simulink model "case2_DCMG_attack_network_detailed_model_R2016"  (R2016a)
settings: Solver=FixedStepDiscrete  SolverMode=SingleTasking  StartTime=0.0  StopTime=3.5  FixedStep=Ts  RelTol=1e-3
InitFcn:
  | Ts=10e-6;
  | R1=0.5;
  | R2=0.6;
  | RD1=4;
  | RD2=4;
  | Vdc1=350;
  | Vdc2=350;
  | Vdcmg_ref=125;
  | Vc1_ref=125;
  | Vc2_ref=125;
model workspace (MAT data in the model file):
  Hamed_Najafi = 1
undefined symbols (not defined in the file): powergui, spspowerguiLib
libraries: powerlib x37, neural x15, simulink x6, powerlib_meascontrol x1
(part 1 of 2)
settings Model: Creator=Aminsystem  LastModifiedBy=Aminsystem
settings DataIOCC: SaveOutput=off  SignalLogging=off  DSMLogging=off  SaveTime=off
settings DebuggingCC: UnconnectedInputMsg=none  UnconnectedOutputMsg=none  UnconnectedLineMsg=none  SFUnexpectedBacktrackingDiag=error  SFNoUnconditionalDefaultTransitionDiag=error
settings ModelReferenceCC: EnableRefExpFcnMdlSchedulingChecks=off
settings SFSimCC: SimUseLocalCustomCode=on
settings RTWCC: Description=Generic Real-Time Target  RTWUseLocalCustomCode=on
settings GRTTargetCC: TargetLangStandard=C99 (ISO)
settings ConfigComp: CovMetricSettings=dwe  CovSaveCumulativeToWorkspaceVar=off  CovSaveSingleToWorkspaceVar=off  CovExternalEMLEnable=on

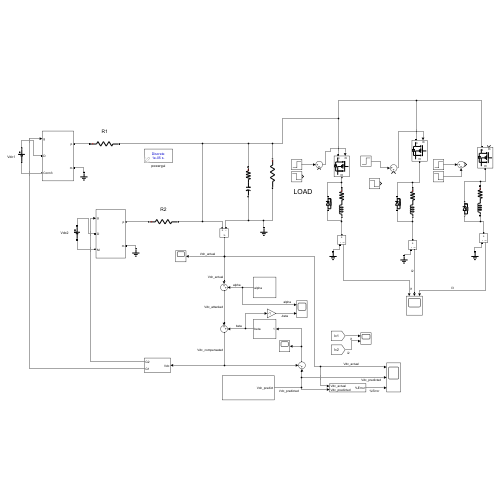
[thumbnail: Simulink's stored preview of the top-level diagram]
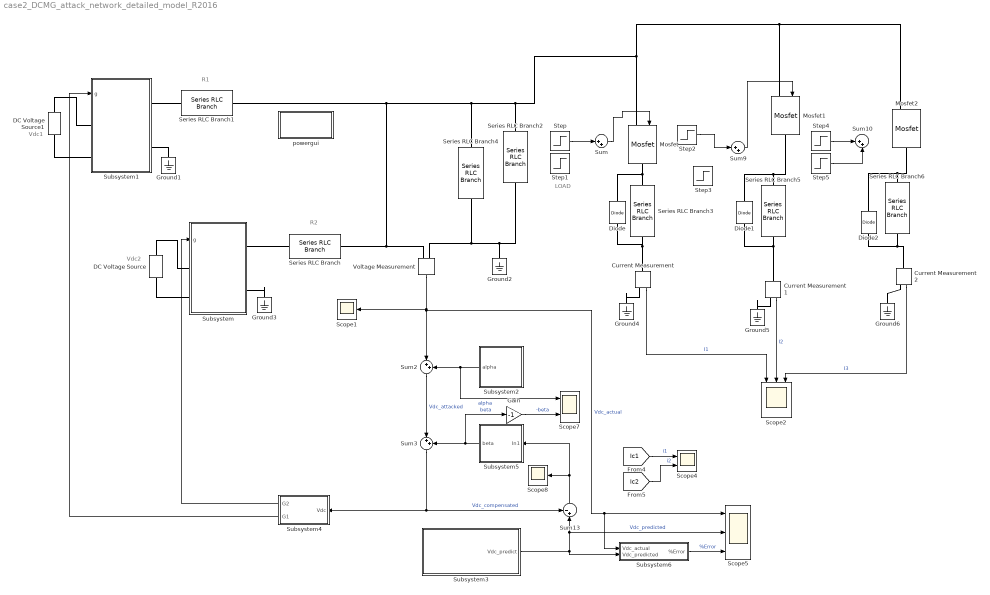
== system case2_DCMG_attack_network_detailed_model_R2016 ==
  note: Vdc2
  note: R2
  note: LOAD
  note: R1
  note: Vdc1
  Current Measurement : powerlib/Measurements/Current Measurement  PhasorSimulation=off  OutputType=Complex  PSBequivalent=0
  Current Measurement1 : powerlib/Measurements/Current Measurement  PhasorSimulation=off  OutputType=Complex  PSBequivalent=0
  Current Measurement2 : powerlib/Measurements/Current Measurement  PhasorSimulation=off  OutputType=Complex  PSBequivalent=0
  DC Voltage Source : powerlib/Electrical Sources/DC Voltage Source  Amplitude=Vdc2  Measurements=None
  DC Voltage Source1 : powerlib/Electrical Sources/DC Voltage Source  Amplitude=Vdc1  Measurements=None
  Diode : powerlib/Power Electronics/Diode  Ron=0.001  Lon=0  Vf=0.8  IC=0  UseSnubber=0  Rs=500  Cs=250e-9  Measurements=off
  Diode1 : powerlib/Power Electronics/Diode  Ron=0.001  Lon=0  Vf=0.8  IC=0  UseSnubber=0  Rs=500  Cs=250e-9  Measurements=off
  Diode2 : powerlib/Power Electronics/Diode  Ron=0.001  Lon=0  Vf=0.8  IC=0  UseSnubber=0  Rs=500  Cs=250e-9  Measurements=off
  Gain : Gain  Gain=-1
  Ground{1..6} (6 alike) : powerlib/Elements/Ground  LConnTagsString=a
  Mosfet : powerlib/Power Electronics/Mosfet  Ron=0.1  Lon=0  Rd=0.01  Vfd=0  IC=0  Rs=1e5  Cs=inf  Measurements=off
  Mosfet1 : powerlib/Power Electronics/Mosfet  Ron=0.1  Lon=0  Rd=0.01  Vfd=0  IC=0  Rs=1e5  Cs=inf  Measurements=off
  Mosfet2 : powerlib/Power Electronics/Mosfet  Ron=0.1  Lon=0  Rd=0.01  Vfd=0  IC=0  Rs=1e5  Cs=inf  Measurements=off
  Scope1 : Scope
  Scope2 : Scope  NumInputPorts=3
  Scope4 : Scope  NumInputPorts=2
  Scope5 : Scope  NumInputPorts=3
  Scope7 : Scope  NumInputPorts=2
  Scope8 : Scope
  Series RLC Branch : powerlib/Elements/Series RLC Branch  LConnTagsString=__new0  RConnTagsString=__new0  BranchType=R  Resistance=R2  Inductance=1e-3  SetiL0=off  InitialCurrent=0  Capacitance=1e-6  Setx0=off  InitialVoltage=0  Measurements=None
  Series RLC Branch1 : powerlib/Elements/Series RLC Branch  LConnTagsString=__new0  RConnTagsString=__new0  BranchType=R  Resistance=R1  Inductance=1e-3  SetiL0=off  InitialCurrent=0  Capacitance=1e-6  Setx0=off  InitialVoltage=0  Measurements=None
  Series RLC Branch2 : powerlib/Elements/Series RLC Branch  LConnTagsString=__new0  RConnTagsString=__new0  BranchType=R  Resistance=60  Inductance=1e-3  SetiL0=off  InitialCurrent=0  Capacitance=1e-6  Setx0=off  InitialVoltage=0  Measurements=None
  Series RLC Branch3 : powerlib/Elements/Series RLC Branch  LConnTagsString=__new0  RConnTagsString=__new0  BranchType=RL  Resistance=60  Inductance=2e-3  SetiL0=off  InitialCurrent=0  Capacitance=1e-6  Setx0=off  InitialVoltage=0  Measurements=None
  Series RLC Branch4 : powerlib/Elements/Series RLC Branch  LConnTagsString=__new0  RConnTagsString=__new0  BranchType=RC  Resistance=0.01  Inductance=1e-3  SetiL0=off  InitialCurrent=0  Capacitance=100e-6  Setx0=on  InitialVoltage=125  Measurements=None
  Series RLC Branch5 : powerlib/Elements/Series RLC Branch  LConnTagsString=__new0  RConnTagsString=__new0  BranchType=RL  Resistance=120  Inductance=5e-3  SetiL0=off  InitialCurrent=0  Capacitance=1e-6  Setx0=off  InitialVoltage=0  Measurements=None
  Series RLC Branch6 : powerlib/Elements/Series RLC Branch  LConnTagsString=__new0  RConnTagsString=__new0  BranchType=RL  Resistance=1.5  Inductance=10e-3  SetiL0=off  InitialCurrent=0  Capacitance=1e-6  Setx0=off  InitialVoltage=0  Measurements=None
  Step : Step  Time=0.5  SampleTime=Ts
  Step1 : Step  Time=2.3  After=-1  SampleTime=Ts
  Step2 : Step  Time=2.5  SampleTime=Ts
  Step3 : Step  Time=3.5  After=-1  SampleTime=Ts
  Step4 : Step  Time=4  SampleTime=Ts
  Step5 : Step  Time=4.2  After=-1  SampleTime=Ts
  Subsystem : Subsystem
  Subsystem1 : Subsystem
  Subsystem2 : Subsystem
  Subsystem3 : Subsystem
  Subsystem4 : Subsystem
  Subsystem5 : Subsystem
  Subsystem6 : Subsystem
  Sum{,2..3,9..10} (5 alike) : Sum  Inputs=|++
  Sum13 : Sum  Inputs=-+|
  Voltage Measurement : powerlib/Measurements/Voltage Measurement  PhasorSimulation=off  OutputType=Complex  PSBequivalent=0
  powergui : Subsystem  Priority=1  AncestorBlock=spspowerguiLib/powergui  DialogController=POWERSYS.PowerSysDialog  InitFcn=powergui( 'InitFcn_Callback' , gcb , 0 , [ ] );  mask(PSB option menu block){SimulationMode=Discrete, SampleTime=Ts, frequency=60, Iterations=50, frequencyindice=0, Pbase=100e6, ErrMax=1e-4, UnitsV=kV, UnitsW=MW, buscounter=0, FunctionMessages=off, echomessages=off, EnableUseOfTLC=off, CurrentSourceSwitches=off, DisableSnubberDevices=off, DisableRonSwitches=off, DisableVfSwitches=off, DisplayEquations=off, AutomaticDiscreteSolvers=off, SolverType=Tustin/Backward Euler (TBE), Interpol=off, ExternalGateDelay=off, methode=off, Ts=100, x0status=blocks, SPID=on, SwTol=0, HookPort=off, NonlinearTolerance=1e-4, nMaxIteration=100, ContinueOnMaxIteration=off, RestoreLinks=warning, ResistiveCurrentMeasurement=off, Frange=[0:2:500], Ylog=off, Xlog=on, ShowGrid=off, save=off, variable=ZData, structure=0, ZoomFFT=off, StartTime=0.0, cycles=1, DisplayStyle=1, fundamental=60, FreqAxis=off, MaxFrequency=1000, frequencyindicesteady=1, RmsSteady=1, display=off}
      mask prompts: SimulationMode "Simulation type:"; SampleTime "Sample time (s):"; frequency "Frequency (Hz):"; Iterations "Max iterations"; frequencyindice "Frequency (Hz)"; Pbase "Base power (VA)"; ErrMax "PQ tolerance (pu)"; UnitsV "Voltage units"; UnitsW "Power units"; buscounter "Load flow bus counter"; FunctionMessages "Disable Specialized Power Systems warnings"; echomessages "Display Specialized Power Systems compilation messages"; EnableUseOfTLC "Use TLC file when in Accelerator Simulation Mode and for code generation"; CurrentSourceSwitches "Disable ideal switching"; DisableSnubberDevices "Disable snubbers in switching devices"; DisableRonSwitches "Disable Ron resistances in switching devices"; DisableVfSwitches "Disable forward voltages in switching devices"; DisplayEquations "Display circuit differential equations"; AutomaticDiscreteSolvers "Automatically handle Discrete solver and Advanced tab solver settings of blocks"; SolverType "Discrete solver"; Interpol "Interpolate switching events"; ExternalGateDelay "Use time-stamped gate signals"; methode "Store switching topologies"; Ts "Buffer size (MBytes):"; x0status "Start simulation with initial electrical states from:"; SPID "Use ideal switching devices"; SwTol "Switch tolerance"; HookPort "Allow multiple powergui blocks"; NonlinearTolerance "Solver tolerance"; nMaxIteration "Maximum number of iterations"; ContinueOnMaxIteration "Continue Simulation if maximum number of iterations is reached"; RestoreLinks "Restore disabled links of Simscape Power Systems ST blocks:"; ResistiveCurrentMeasurement "Use non ideal current measurement blocks (1e-4Ohm internal resistance)"; Frange "Frequency Range"; Ylog "Log impedance"; Xlog "log Frequency"; ShowGrid "grid"; save "Save Data To Workspace"; variable "Variable Name"; structure "Structure Name (PSBFFTSCOPE)"; ZoomFFT "ZoomFFT (PSBFFTSCOPE)"; StartTime "Start Time (PSBFFTSCOPE)"; cycles "Cycles (PSBFFTSCOPE)"; DisplayStyle "Display style (PSBFFTSCOPE)"; fundamental "Fundamental (PSBFFTSCOPE)"; FreqAxis "Frequency Axis (PSBFFTSCOPE)"; MaxFrequency "Max Frequency (PSBFFTSCOPE)"; frequencyindicesteady "Frequency indice (STEADYSTATE)"; RmsSteady "RMS display (STEADYSTATE)"; display "Display Results"
      mask help: Set simulation type, simulation parameters, and preferences.
      mask init:
      | dispMessage = '';
      | dispMessage = powergui('MaskInitialization',gcb,SimulationMode,SampleTime);
      settings: PreSaveFcn=powergui( 'PreSaveFcn_Callback' , gcb , [ ] , [ ] );  OpenFcn=sps_rtmsupport('OpenFcn',gcbh)
      mask Help: helpview(psbhelp)
      mask TypeOptions SimulationMode: Continuous | Discrete | Phasor | Discrete phasor
      mask Callback SimulationMode: powergui('SimulationType',[],[],gcb);
      mask TypeOptions UnitsV: V | kV
      mask TypeOptions UnitsW: W | kW | MW
      mask Callback CurrentSourceSwitches: powergui('SimulationType',[],[],gcb);
      mask Callback AutomaticDiscreteSolvers: powergui('SimulationType',[],[],gcb);
      mask TypeOptions SolverType: Tustin/Backward Euler (TBE) | Tustin | Backward Euler
      mask Callback SolverType: powergui('SimulationType',[],[],gcb);
      mask Callback Interpol: powergui('SimulationType',[],[],gcb);
      mask Callback ExternalGateDelay: powergui('SimulationType',[],[],gcb);
      mask Callback methode: powergui('SimulationType',[],[],gcb);
      mask TypeOptions x0status: blocks | steady | zero
      mask TypeOptions RestoreLinks: yes | warning | no
      mask Callback display: sps_rtmsupport('parametereditingmodes',gcbh) % Will be executed last in parameter callbacks to ensure mask enable consistency
      mask DialogControl AutoSolverNote Prompt: The Simulation type parameter is governed by Simulink. To access the Powergui solver settings, unselect auto (Automatic solver selection) solver in the Simulink solver options.
      mask DialogControl StateAnalyzer Prompt: Measurements and States Analyzer
      mask DialogControl StateAnalyzer Callback: powerStates(bdroot(gcb))
      mask DialogControl LineParameterCalculator Prompt: Line Parameter Calculator
      mask DialogControl LineParameterCalculator Callback:
      | close_system(gcb)
      | powerLineParameters
      mask DialogControl CableParameterCalculator Prompt: Cable Parameter Calculator
      mask DialogControl CableParameterCalculator Callback:
      | close_system(gcb)
      | powerCableParameters
      mask DialogControl LineDecoupler Prompt: Line Decoupler
      mask DialogControl LineDecoupler Tooltip: Click to replace selected Distributed Parameters Line blocks with Decoupling Line blocks
      mask DialogControl LineDecoupler Callback:
      | close_system(gcb);
      | DecouplingLineReplace(gcs)
      mask DialogControl LoadFlowAnalyzer Prompt: Load Flow Analyzer
      mask DialogControl LoadFlowAnalyzer Callback:
      | close_system(gcb)
      | powerLoadFlow
      mask DialogControl LoadFlowParameters Prompt: Load Flow Parameters
      mask DialogControl ImpedanceCalculator Prompt: Impedance Calculator
      mask DialogControl ImpedanceCalculator Callback:
      | close_system(gcb);
      | powerImpedance(bdroot(gcs));
      mask DialogControl FFTAnalyzer Prompt: FFT Analyzer
      mask DialogControl FFTAnalyzer Callback:
      | close_system(gcb)
      | power_fftscope(bdroot(gcb),gcb)
      mask DialogControl LinearSystemAnalyzer Prompt: Linear System Analyzer
      mask DialogControl LinearSystemAnalyzer Callback:
      | close_system(gcb)
      | power_ltiview(bdroot(gcb))
      mask DialogControl HysteresisDesigner Prompt: Hysteresis Designer
      mask DialogControl HysteresisDesigner Callback:
      | close_system(gcb)
      | powerHysteresis('hysteresis.mat')
      mask DialogControl BlockCustomizer Prompt: Block Customizer
      mask DialogControl BlockCustomizer Callback:
      | close_system(gcb);
      | power_customize;
      mask DialogControl ReportGenerator Prompt: Report Generator
      mask DialogControl ReportGenerator Callback:
      | close_system(gcb)
      | power_report(bdroot(gcb))
      mask DialogControl obsolete Prompt: ...
      mask DialogControl MachineInitialization Prompt: Machine Initialization
      mask DialogControl MachineInitialization Callback:
      | close_system(gcb)
      | powericon('machineInitTool',bdroot(gcb),gcb)
      mask DialogControl Solver Prompt: Solver
      mask DialogControl SolverDetails Prompt: Solver details for nonlinear elements
      mask Display: color('blue'),disp(dispMessage)
  wires:
  Sum3/1 -> Sum13/1, Subsystem4/1(Vdc)  "Vdc_compensated"
  Step/1 -> Sum/1
  Sum/1 -> Mosfet/1
  Step2/1 -> Sum9/1
  Step4/1 -> Sum10/1
  Step5/1 -> Sum10/2
  Current Measurement/1 -> Scope2/1  "I1"
  Current Measurement1/1 -> Scope2/2  "I2"
  Current Measurement2/1 -> Scope2/3  "I3"
  Sum9/1 -> Mosfet1/1
  Voltage Measurement/1 -> Sum2/1, Scope5/1, Subsystem6/1(Vdc_actual), Scope1/1  "Vdc_actual"
  Sum13/1 -> Subsystem5/1(In1), Scope8/1
  [Ic1] -> Scope4/1  "i1"
  [Ic2] -> Scope4/2  "i2"
  Subsystem3/1(Vdc_predict) -> Scope5/2, Sum13/2, Subsystem6/2(Vdc_predicted)  "Vdc_predicted"
  Sum2/1 -> Sum3/1  "Vdc_attacked"
  Subsystem4/2(G1) -> Subsystem1/1(g)
  Subsystem4/1(G2) -> Subsystem/1(g)
  Subsystem2/1(alpha) -> Sum2/2, Scope7/1  "alpha"
  Subsystem5/1(beta) -> Gain/1, Sum3/2  "beta"
  Subsystem6/1(%Error) -> Scope5/3  "%Error"
  Gain/1 -> Scope7/2  "-beta"
  connections:
  Series RLC Branch5/RConn1 -- Diode1/LConn1 -- Current Measurement1/LConn1
  Series RLC Branch2/LConn1 -- Mosfet/LConn1 -- Mosfet2/LConn1 -- Mosfet1/LConn1 -- Series RLC Branch4/LConn1 -- Series RLC Branch1/RConn1 -- Series RLC Branch/RConn1 -- Voltage Measurement/LConn1
  Mosfet/RConn1 -- Diode/RConn1 -- Series RLC Branch3/LConn1
  Series RLC Branch3/RConn1 -- Diode/LConn1 -- Current Measurement/LConn1
  Voltage Measurement/LConn2 -- Ground2/LConn1 -- Series RLC Branch2/RConn1 -- Series RLC Branch4/RConn1
  Current Measurement2/LConn1 -- Diode2/LConn1 -- Series RLC Branch6/RConn1
  Series RLC Branch5/LConn1 -- Mosfet1/RConn1 -- Diode1/RConn1
  Diode2/RConn1 -- Mosfet2/RConn1 -- Series RLC Branch6/LConn1
  Series RLC Branch/LConn1 -- Subsystem/RConn1
  Subsystem/LConn1 -- DC Voltage Source/RConn1
  DC Voltage Source/LConn1 -- Subsystem/LConn2
  Series RLC Branch1/LConn1 -- Subsystem1/RConn1
  Subsystem1/LConn1 -- DC Voltage Source1/RConn1
  Subsystem1/LConn2 -- DC Voltage Source1/LConn1
  Ground1/LConn1 -- Subsystem1/RConn2
  Ground3/LConn1 -- Subsystem/RConn2
  Ground4/LConn1 -- Current Measurement/RConn1
  Ground5/LConn1 -- Current Measurement1/RConn1
  Ground6/LConn1 -- Current Measurement2/RConn1

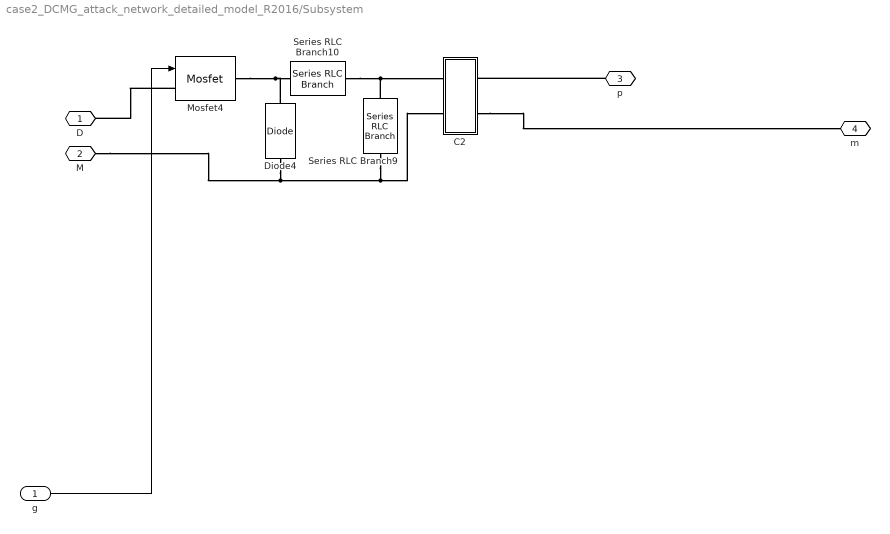
== system case2_DCMG_attack_network_detailed_model_R2016/Subsystem ==
  g : Inport
  C2 : Subsystem
  Diode4 : powerlib/Power Electronics/Diode  Ron=0.001  Lon=0  Vf=0.8  IC=0  UseSnubber=0  Rs=500  Cs=250e-9  Measurements=off
  Mosfet4 : powerlib/Power Electronics/Mosfet  Ron=0.1  Lon=0  Rd=0.01  Vfd=0  IC=0  Rs=1e5  Cs=inf  Measurements=off
  Series RLC Branch10 : powerlib/Elements/Series RLC Branch  LConnTagsString=__new0  RConnTagsString=__new0  BranchType=L  Resistance=0.01  Inductance=50e-3  SetiL0=off  InitialCurrent=0  Capacitance=57e-6  Setx0=off  InitialVoltage=120  Measurements=None
  Series RLC Branch9 : powerlib/Elements/Series RLC Branch  LConnTagsString=__new0  RConnTagsString=__new0  BranchType=C  Resistance=0.01  Inductance=1e-3  SetiL0=off  InitialCurrent=0  Capacitance=50e-6  Setx0=on  InitialVoltage=125  Measurements=None
  D : PMIOPort  Side=Left
  M : PMIOPort  Port=2  Side=Left
  p : PMIOPort  Port=3  Side=Right
  m : PMIOPort  Port=4  Side=Right
  wires:
  g/1 -> Mosfet4/1
  connections:
  Diode4/RConn1 -- Mosfet4/RConn1 -- Series RLC Branch10/RConn1
  Mosfet4/LConn1 -- D/RConn1
  Series RLC Branch9/LConn1 -- Series RLC Branch10/LConn1 -- C2/LConn1
  Diode4/LConn1 -- M/RConn1 -- Series RLC Branch9/RConn1 -- C2/LConn2
  p/RConn1 -- C2/RConn1
  C2/RConn2 -- m/RConn1

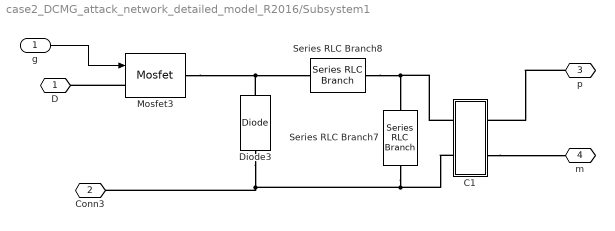
== system case2_DCMG_attack_network_detailed_model_R2016/Subsystem1 ==
  g : Inport
  C1 : Subsystem
  Diode3 : powerlib/Power Electronics/Diode  Ron=0.001  Lon=0  Vf=0.8  IC=0  UseSnubber=0  Rs=500  Cs=250e-9  Measurements=off
  Mosfet3 : powerlib/Power Electronics/Mosfet  Ron=0.1  Lon=0  Rd=0.01  Vfd=0  IC=0  Rs=1e5  Cs=inf  Measurements=off
  Series RLC Branch7 : powerlib/Elements/Series RLC Branch  LConnTagsString=__new0  RConnTagsString=__new0  BranchType=C  Resistance=0.01  Inductance=1e-3  SetiL0=off  InitialCurrent=0  Capacitance=50e-6  Setx0=on  InitialVoltage=125  Measurements=None
  Series RLC Branch8 : powerlib/Elements/Series RLC Branch  LConnTagsString=__new0  RConnTagsString=__new0  BranchType=L  Resistance=0.01  Inductance=50e-3  SetiL0=off  InitialCurrent=0  Capacitance=57e-6  Setx0=off  InitialVoltage=120  Measurements=None
  D : PMIOPort  Side=Left
  Conn3 : PMIOPort  Port=2  Side=Left
  p : PMIOPort  Port=3  Side=Right
  m : PMIOPort  Port=4  Side=Right
  wires:
  g/1 -> Mosfet3/1
  connections:
  C1/LConn2 -- Conn3/RConn1 -- Diode3/LConn1 -- Series RLC Branch7/RConn1
  Diode3/RConn1 -- Mosfet3/RConn1 -- Series RLC Branch8/RConn1
  Mosfet3/LConn1 -- D/RConn1
  Series RLC Branch8/LConn1 -- C1/LConn1 -- Series RLC Branch7/LConn1
  C1/RConn2 -- m/RConn1
  p/RConn1 -- C1/RConn1

== system case2_DCMG_attack_network_detailed_model_R2016/Subsystem2 ==
  Sine Wave Function : Sin  Amplitude=10  Frequency=2*pi*1  SampleTime=Ts
  Step8 : Step  Time=0.5  SampleTime=Ts
  Switch : Switch  Criteria=u2 > Threshold
  Zero : Constant  Value=0  OutDataTypeStr=Inherit: Inherit via back propagation
  alpha : Outport
  wires:
  Switch/1 -> alpha/1  "alpha"
  Step8/1 -> Switch/2
  Zero/1 -> Switch/3
  Sine Wave Function/1 -> Switch/1

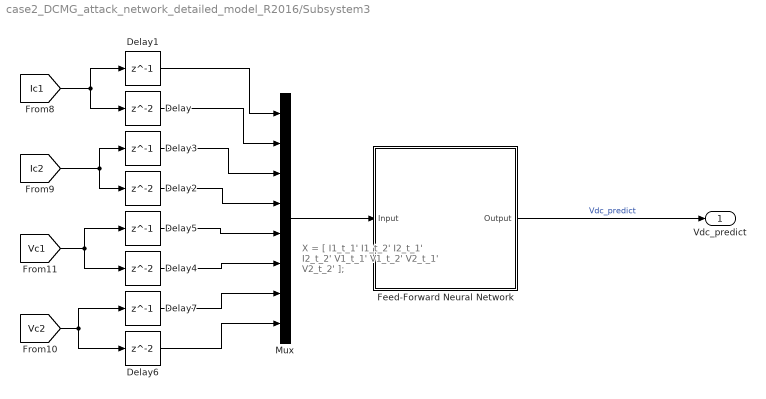
== system case2_DCMG_attack_network_detailed_model_R2016/Subsystem3 ==
  note: X = [
      | I1_t_1'
      | I1_t_2'
      | I2_t_1'
      | I2_t_2'
      | V1_t_1'
      | V1_t_2'
      | V2_t_1'
      | V2_t_2'
      | ];
  Delay{,2,4,6} (4 alike) : Delay  SampleTime=Ts
  Delay{1,3,5,7} (4 alike) : Delay  DelayLength=1  SampleTime=Ts
  Feed-Forward Neural Network : Subsystem
      mask help: Feed-Forward Neural Network
      mask Display: e = 0.06;c1 = [120 150 230]/255;c2 = ([120 150 230]+0)/383;c3 = ([120 150 230]+128)/383;patch([0 1 1 0],[0 0 1 1],c1);patch([0 1 1 1-e 1-e 0+e],[0 0 1 1-e 0+e 0+e],c2);patch([0 0 1 1-e 0+e 0+e],[0 1 1 1-e 1-e 0+e],c3);plot([0 1 1 0 0],[0 0 1 1 0]);fprintf('NNET');port_label('input',1,' Input');port_label('output',1,'Output ');
  Mux : Mux  Inputs=8
  Vdc_predict : Outport
  wires:
  Delay3/1 -> Mux/3
  [Ic1] -> Delay1/1, Delay/1
  [Ic2] -> Delay3/1, Delay2/1
  Feed-Forward Neural Network/1(Output) -> Vdc_predict/1  "Vdc_predict"
  Delay/1 -> Mux/2
  Delay4/1 -> Mux/6
  Delay6/1 -> Mux/8
  Mux/1 -> Feed-Forward Neural Network/1(Input)
  Delay5/1 -> Mux/5
  [Vc2] -> Delay7/1, Delay6/1
  [Vc1] -> Delay5/1, Delay4/1
  Delay2/1 -> Mux/4
  Delay7/1 -> Mux/7
  Delay1/1 -> Mux/1

== system case2_DCMG_attack_network_detailed_model_R2016/Subsystem4 ==
  note: V*dc
  Vdc : Inport
  Subsystem2 : Subsystem
  Sum1 : Sum  Inputs=-+|
  Zero2 : Constant  Value=Vdcmg_ref  OutDataTypeStr=Inherit: Inherit via back propagation  SampleTime=Ts
  G2 : Outport
  G1 : Outport  Port=2
  wires:
  Vdc/1 -> Sum1/1
  Zero2/1 -> Sum1/2
  Subsystem2/1(P) -> G1/1
  Subsystem2/2(Out2) -> G2/1
  Sum1/1 -> Subsystem2/1(u)

== system case2_DCMG_attack_network_detailed_model_R2016/Subsystem5 ==
  In1 : Inport
  PID Controller5 : simulink/Continuous/PID Controller  Controller=PI  Form=Parallel  TimeDomain=Discrete-time  SampleTime=Ts  IntegratorMethod=Forward Euler  FilterMethod=Forward Euler  ControllerParametersSource=internal  P=0.2*0+20  I=1*0+100  D=0  N=100  UseFilter=on  InitialConditionSource=internal  InitialConditionForIntegrator=0  InitialConditionForFilter=0  DifferentiatorICPrevScaledInput=0  ExternalReset=none  TrackingMode=off  Kt=1  LimitOutput=off  UpperSaturationLimit=inf  LowerSaturationLimit=-inf  LinearizeAsGain=on  AntiWindupMode=none  Kb=1  POutMin=[]  POutMax=[]  IOutMin=[]  IOutMax=[]  DOutMin=[]  DOutMax=[]  NOutMin=[]  NOutMax=[]  SumOutMin=[]  SumOutMax=[]  SaturationOutMin=[]  SaturationOutMax=[]  PParamMin=[]  PParamMax=[]  IParamMin=[]  IParamMax=[]  DParamMin=[]  DParamMax=[]  NParamMin=[]  NParamMax=[]  KbParamMin=[]  KbParamMax=[]  KtParamMin=[]  KtParamMax=[]  KbOutMin=[]  KbOutMax=[]  KtOutMin=[]  KtOutMax=[]  IntegratorOutMin=[]  IntegratorOutMax=[]  FilterOutMin=[]  FilterOutMax=[]  SumI1OutMin=[]  SumI1OutMax=[]  SumI2OutMin=[]  SumI2OutMax=[]  SumI3OutMin=[]  SumI3OutMax=[]  SumDOutMin=[]  SumDOutMax=[]  DifferentiatorOutMin=[]  DifferentiatorOutMax=[]  IntegratorContinuousStateAttributes=''  IntegratorStateMustResolveToSignalObject=off  IntegratorRTWStateStorageClass=Auto  FilterContinuousStateAttributes=''  FilterStateMustResolveToSignalObject=off  FilterRTWStateStorageClass=Auto
  Step8 : Step  Time=0.01  SampleTime=Ts
  Switch : Switch  Criteria=u2 > Threshold
  Zero : Constant  Value=0  OutDataTypeStr=Inherit: Inherit via back propagation
  beta : Outport
  wires:
  Zero/1 -> Switch/3
  Switch/1 -> PID Controller5/1
  Step8/1 -> Switch/2
  PID Controller5/1 -> beta/1  "beta"
  In1/1 -> Switch/1

== system case2_DCMG_attack_network_detailed_model_R2016/Subsystem6 ==
  Vdc_actual : Inport
  Vdc_predicted : Inport  Port=2
  Divide : Product  Inputs=*/  RndMeth=Zero  SaturateOnIntegerOverflow=on
  Saturation : Saturate  UpperLimit=inf  LowerLimit=1
  Sum11 : Sum  Inputs=+-|
  %Error : Outport
  wires:
  Saturation/1 -> Divide/2
  Sum11/1 -> Divide/1
  Vdc_actual/1 -> Saturation/1, Sum11/1
  Divide/1 -> %Error/1  "%Error"
  Vdc_predicted/1 -> Sum11/2

== system case2_DCMG_attack_network_detailed_model_R2016/powergui ==
  note: Graphical user interface for the analysis of
      | Simscape Power Systems (Specialized Technology) circuits.
      | Place the Powergui block in the top-level of your model and double-click
      | on it to open the GUI.
  EquivalentModel1 : Subsystem
      mask init:
      | S  = GetDataForEquivalentModel('Discrete',gcbh);
      mask Display:
      | color('red')
      | disp('EQUIVALENT CIRCUIT\nDiscrete')
  Ground : Ground
  Terminator : Terminator
  wires:
  Ground/1 -> Terminator/1

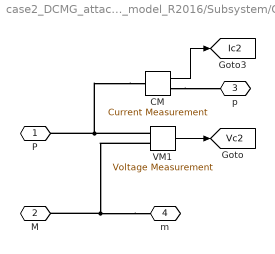
== system case2_DCMG_attack_network_detailed_model_R2016/Subsystem/C2 ==
  CM : powerlib/Measurements/Current Measurement  PhasorSimulation=off  OutputType=Complex  PSBequivalent=0
  VM1 : powerlib/Measurements/Voltage Measurement  PhasorSimulation=off  OutputType=Complex  PSBequivalent=0
  P : PMIOPort  Side=Left
  M : PMIOPort  Port=2  Side=Left
  p : PMIOPort  Port=3  Side=Right
  m : PMIOPort  Port=4  Side=Right
  tag scope: Ic2=global, Vc2=global
  wires:
  CM/1 -> [Ic2]
  VM1/1 -> [Vc2]
  connections:
  CM/RConn1 -- p/RConn1
  m/RConn1 -- VM1/LConn2 -- M/RConn1
  CM/LConn1 -- VM1/LConn1 -- P/RConn1

== system case2_DCMG_attack_network_detailed_model_R2016/Subsystem1/C1 ==
  CM : powerlib/Measurements/Current Measurement  PhasorSimulation=off  OutputType=Complex  PSBequivalent=0
  VM1 : powerlib/Measurements/Voltage Measurement  PhasorSimulation=off  OutputType=Complex  PSBequivalent=0
  P : PMIOPort  Side=Left
  M : PMIOPort  Port=2  Side=Left
  p : PMIOPort  Port=3  Side=Right
  m : PMIOPort  Port=4  Side=Right
  tag scope: Ic1=global, Vc1=global
  wires:
  VM1/1 -> [Vc1]
  CM/1 -> [Ic1]
  connections:
  P/RConn1 -- VM1/LConn1 -- CM/LConn1
  M/RConn1 -- VM1/LConn2 -- m/RConn1
  CM/RConn1 -- p/RConn1

== system case2_DCMG_attack_network_detailed_model_R2016/Subsystem3/Feed-Forward Neural Network ==
  Input : Inport  PortDimensions=8
      mask Display: e = 0.06;c1 = [120 230 180]/255;c2 = ([120 230 180]+0)/(256+128);c3 = ([120 230 180]+128)/(256+128);patch([0 1 1 0],[0 0 1 1],c1);patch([0 1 1 1-e 1-e 0+e],[0 0 1 1-e 0+e 0+e],c2);patch([0 0 1 1-e 0+e 0+e],[0 1 1 1-e 1-e 0+e],c3);plot([0 1 1 0 0],[0 0 1 1 0]);
  Layer 1 : Subsystem
      mask Display: e = 0.06;c1 = [120 150 230]/255;c2 = ([120 150 230]+0)/383;c3 = ([120 150 230]+128)/383;patch([0 1 1 0],[0 0 1 1],c1);patch([0 1 1 1-e 1-e 0+e],[0 0 1 1-e 0+e 0+e],c2);patch([0 0 1 1-e 0+e 0+e],[0 1 1 1-e 1-e 0+e],c3);plot([0 1 1 0 0],[0 0 1 1 0]);
  Layer 2 : Subsystem
      mask Display: e = 0.06;c1 = [120 150 230]/255;c2 = ([120 150 230]+0)/383;c3 = ([120 150 230]+128)/383;patch([0 1 1 0],[0 0 1 1],c1);patch([0 1 1 1-e 1-e 0+e],[0 0 1 1-e 0+e 0+e],c2);patch([0 0 1 1-e 0+e 0+e],[0 1 1 1-e 1-e 0+e],c3);plot([0 1 1 0 0],[0 0 1 1 0]);
  Process Input 1 : Subsystem
      mask Display: e = 0.06;c1 = [120 150 230]/255;c2 = ([120 150 230]+0)/383;c3 = ([120 150 230]+128)/383;patch([0 1 1 0],[0 0 1 1],c1);patch([0 1 1 1-e 1-e 0+e],[0 0 1 1-e 0+e 0+e],c2);patch([0 0 1 1-e 0+e 0+e],[0 1 1 1-e 1-e 0+e],c3);plot([0 1 1 0 0],[0 0 1 1 0]);
  Process Output 1 : Subsystem
      mask Display: e = 0.06;c1 = [120 150 230]/255;c2 = ([120 150 230]+0)/383;c3 = ([120 150 230]+128)/383;patch([0 1 1 0],[0 0 1 1],c1);patch([0 1 1 1-e 1-e 0+e],[0 0 1 1-e 0+e 0+e],c2);patch([0 0 1 1-e 0+e 0+e],[0 1 1 1-e 1-e 0+e],c3);plot([0 1 1 0 0],[0 0 1 1 0]);
  Output : Outport  InitialOutput=0
      mask Display: e = 0.06;c1 = [120 230 180]/255;c2 = ([120 230 180]+0)/(256+128);c3 = ([120 230 180]+128)/(256+128);patch([0 1 1 0],[0 0 1 1],c1);patch([0 1 1 1-e 1-e 0+e],[0 0 1 1-e 0+e 0+e],c2);patch([0 0 1 1-e 0+e 0+e],[0 1 1 1-e 1-e 0+e],c3);plot([0 1 1 0 0],[0 0 1 1 0]);
  wires:
  Input/1 -> Process Input 1/1(x)
  Process Output 1/1(y) -> Output/1
  Process Input 1/1(p) -> Layer 1/1("p{1}")
  Layer 1/1("a{1}") -> [feedback1]
  [feedback1] -> Layer 2/1("a{1} ")
  Layer 2/1("a{2}") -> Process Output 1/1(a)

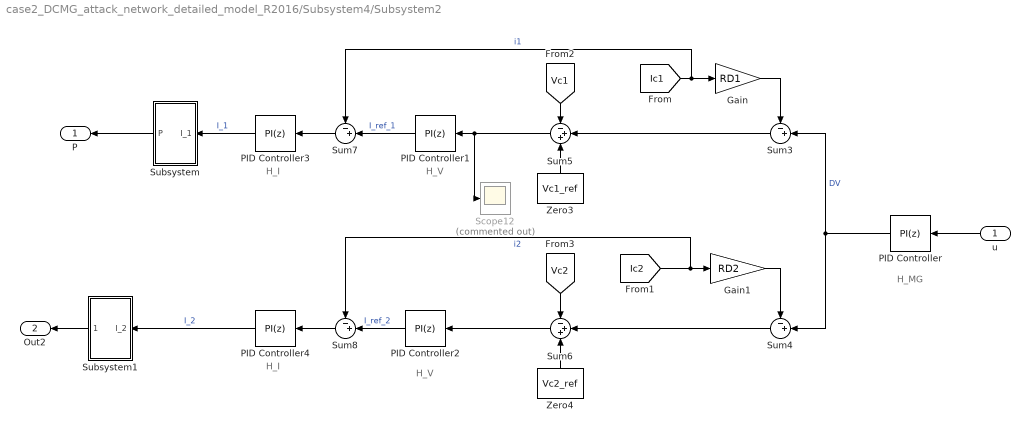
== system case2_DCMG_attack_network_detailed_model_R2016/Subsystem4/Subsystem2 ==
  note: H_V
  note: H_V
  note: H_I
  note: H_I
  note: H_MG
  u : Inport
  Gain : Gain  Gain=RD1
  Gain1 : Gain  Gain=RD2
  PID Controller : simulink/Continuous/PID Controller  Controller=PI  Form=Parallel  TimeDomain=Discrete-time  SampleTime=Ts  IntegratorMethod=Forward Euler  FilterMethod=Forward Euler  ControllerParametersSource=internal  P=1*0+0.5*0+1  I=100  D=0  N=100  UseFilter=on  InitialConditionSource=internal  InitialConditionForIntegrator=0  InitialConditionForFilter=0  DifferentiatorICPrevScaledInput=0  ExternalReset=none  TrackingMode=off  Kt=1  LimitOutput=off  UpperSaturationLimit=inf  LowerSaturationLimit=-inf  LinearizeAsGain=on  AntiWindupMode=none  Kb=1  POutMin=[]  POutMax=[]  IOutMin=[]  IOutMax=[]  DOutMin=[]  DOutMax=[]  NOutMin=[]  NOutMax=[]  SumOutMin=[]  SumOutMax=[]  SaturationOutMin=[]  SaturationOutMax=[]  PParamMin=[]  PParamMax=[]  IParamMin=[]  IParamMax=[]  DParamMin=[]  DParamMax=[]  NParamMin=[]  NParamMax=[]  KbParamMin=[]  KbParamMax=[]  KtParamMin=[]  KtParamMax=[]  KbOutMin=[]  KbOutMax=[]  KtOutMin=[]  KtOutMax=[]  IntegratorOutMin=[]  IntegratorOutMax=[]  FilterOutMin=[]  FilterOutMax=[]  SumI1OutMin=[]  SumI1OutMax=[]  SumI2OutMin=[]  SumI2OutMax=[]  SumI3OutMin=[]  SumI3OutMax=[]  SumDOutMin=[]  SumDOutMax=[]  DifferentiatorOutMin=[]  DifferentiatorOutMax=[]  IntegratorContinuousStateAttributes=''  IntegratorStateMustResolveToSignalObject=off  IntegratorRTWStateStorageClass=Auto  FilterContinuousStateAttributes=''  FilterStateMustResolveToSignalObject=off  FilterRTWStateStorageClass=Auto
  PID Controller{1..4} (4 alike) : simulink/Continuous/PID Controller  Controller=PI  Form=Parallel  TimeDomain=Discrete-time  SampleTime=Ts  IntegratorMethod=Forward Euler  FilterMethod=Forward Euler  ControllerParametersSource=internal  P=10  I=100  D=0  N=100  UseFilter=on  InitialConditionSource=internal  InitialConditionForIntegrator=0  InitialConditionForFilter=0  DifferentiatorICPrevScaledInput=0  ExternalReset=none  TrackingMode=off  Kt=1  LimitOutput=off  UpperSaturationLimit=inf  LowerSaturationLimit=-inf  LinearizeAsGain=on  AntiWindupMode=none  Kb=1  POutMin=[]  POutMax=[]  IOutMin=[]  IOutMax=[]  DOutMin=[]  DOutMax=[]  NOutMin=[]  NOutMax=[]  SumOutMin=[]  SumOutMax=[]  SaturationOutMin=[]  SaturationOutMax=[]  PParamMin=[]  PParamMax=[]  IParamMin=[]  IParamMax=[]  DParamMin=[]  DParamMax=[]  NParamMin=[]  NParamMax=[]  KbParamMin=[]  KbParamMax=[]  KtParamMin=[]  KtParamMax=[]  KbOutMin=[]  KbOutMax=[]  KtOutMin=[]  KtOutMax=[]  IntegratorOutMin=[]  IntegratorOutMax=[]  FilterOutMin=[]  FilterOutMax=[]  SumI1OutMin=[]  SumI1OutMax=[]  SumI2OutMin=[]  SumI2OutMax=[]  SumI3OutMin=[]  SumI3OutMax=[]  SumDOutMin=[]  SumDOutMax=[]  DifferentiatorOutMin=[]  DifferentiatorOutMax=[]  IntegratorContinuousStateAttributes=''  IntegratorStateMustResolveToSignalObject=off  IntegratorRTWStateStorageClass=Auto  FilterContinuousStateAttributes=''  FilterStateMustResolveToSignalObject=off  FilterRTWStateStorageClass=Auto
  Scope12 : Scope  Commented=on
  Subsystem : Subsystem
  Subsystem1 : Subsystem
  Sum{3..4,7..8} (4 alike) : Sum  Inputs=-+|
  Sum5 : Sum  Inputs=-++
  Sum6 : Sum  Inputs=-++
  Zero3 : Constant  Value=Vc1_ref  OutDataTypeStr=Inherit: Inherit via back propagation  SampleTime=Ts
  Zero4 : Constant  Value=Vc2_ref  OutDataTypeStr=Inherit: Inherit via back propagation
  P : Outport
  Out2 : Outport  Port=2
  wires:
  Sum7/1 -> PID Controller3/1
  [Ic1] -> Gain/1, Sum7/1  "i1"
  Sum4/1 -> Sum6/2
  Zero4/1 -> Sum6/3
  Sum5/1 -> Scope12/1, PID Controller1/1
  u/1 -> PID Controller/1
  PID Controller/1 -> Sum4/2, Sum3/2  "DV"
  Zero3/1 -> Sum5/3
  PID Controller2/1 -> Sum8/2  "I_ref_2"
  Gain/1 -> Sum3/1
  [Vc2] -> Sum6/1
  PID Controller1/1 -> Sum7/2  "I_ref_1"
  [Ic2] -> Sum8/1, Gain1/1  "i2"
  Subsystem/1(P) -> P/1
  Sum8/1 -> PID Controller4/1
  Gain1/1 -> Sum4/1
  Sum3/1 -> Sum5/2
  Sum6/1 -> PID Controller2/1
  PID Controller4/1 -> Subsystem1/1(I_2)  "I_2"
  [Vc1] -> Sum5/1
  PID Controller3/1 -> Subsystem/1(I_1)  "I_1"
  Subsystem1/1(Out1) -> Out2/1

== system case2_DCMG_attack_network_detailed_model_R2016/powergui/EquivalentModel1 ==
  Gates : Subsystem
  Sources : Subsystem
  State-Space : S-Function  FunctionName=sfun_spssw_discc  Parameters=S.Ts,S.A, S.B, S.C, S.D, S.x0, S.EnableUseOfTLC,S.SwitchResistance ,S.SwitchType, S.SwitchGateInitialValue, S.OutputsToResetToZero, S.TBEON,S.SaveMatrices,S.BufferSize  SFunctionDeploymentMode=off  EnableBusSupport=off
  Status : Subsystem
  Yout : Subsystem
  wires:
  Gates/1(gates) -> State-Space/2
  Sources/1(u) -> State-Space/1
  State-Space/2 -> Status/1(status)
  State-Space/1 -> Yout/1(v,i)

== system case2_DCMG_attack_network_detailed_model_R2016/Subsystem3/Feed-Forward Neural Network/Layer 1 ==
  "p{1}" : Inport  PortDimensions=8
      mask Display: e = 0.06;c1 = [120 230 180]/255;c2 = ([120 230 180]+0)/(256+128);c3 = ([120 230 180]+128)/(256+128);patch([0 1 1 0],[0 0 1 1],c1);patch([0 1 1 1-e 1-e 0+e],[0 0 1 1-e 0+e 0+e],c2);patch([0 0 1 1-e 0+e 0+e],[0 1 1 1-e 1-e 0+e],c3);plot([0 1 1 0 0],[0 0 1 1 0]);
  Delays 1 : Subsystem
      mask Display: e = 0.06;c1 = [120 150 230]/255;c2 = ([120 150 230]+0)/383;c3 = ([120 150 230]+128)/383;patch([0 1 1 0],[0 0 1 1],c1);patch([0 1 1 1-e 1-e 0+e],[0 0 1 1-e 0+e 0+e],c2);patch([0 0 1 1-e 0+e 0+e],[0 1 1 1-e 1-e 0+e],c3);plot([0 1 1 0 0],[0 0 1 1 0]);disp('0');
  "IW{1,1}" : Subsystem
      mask Display: e = 0.06;c1 = [120 150 230]/255;c2 = ([120 150 230]+0)/383;c3 = ([120 150 230]+128)/383;patch([0 1 1 0],[0 0 1 1],c1);patch([0 1 1 1-e 1-e 0+e],[0 0 1 1-e 0+e 0+e],c2);patch([0 0 1 1-e 0+e 0+e],[0 1 1 1-e 1-e 0+e],c3);plot([0 1 1 0 0],[0 0 1 1 0]);disp('W');
  "b{1}" : Constant  Value=[1.9984097654395469589871936477720737457275390625;-0.75620084897652362077025145481457002460956573486328125;1.6888107581719549177279304785770364105701446533203125;-0.171277151305295582961463196625118143856525421142578125;0.7279147608841574079718839129782281816005706787109375;0.40153888476495647186226278790854848921298980712890625;0.435876758337768788198474112505209632217884063720703125;1.0865141598479548523670246140682138502597808837890625;0.88654793089141359363480887623154558241367340087890625;-2.151943139408628358211217346251942217350006103515625]
      mask Display: e = 0.06;c1 = [120 150 230]/255;c2 = ([120 150 230]+0)/383;c3 = ([120 150 230]+128)/383;patch([0 1 1 0],[0 0 1 1],c1);patch([0 1 1 1-e 1-e 0+e],[0 0 1 1-e 0+e 0+e],c2);patch([0 0 1 1-e 0+e 0+e],[0 1 1 1-e 1-e 0+e],c3);plot([0 1 1 0 0],[0 0 1 1 0]);disp('b');
  netsum : Sum  Inputs=2  InputSameDT=on  SaturateOnIntegerOverflow=on  OutDataTypeStr=Inherit: Same as first input
      mask Display: e = 0.06;c1 = [120 150 230]/255;c2 = ([120 150 230]+0)/383;c3 = ([120 150 230]+128)/383;patch([0 1 1 0],[0 0 1 1],c1);patch([0 1 1 1-e 1-e 0+e],[0 0 1 1-e 0+e 0+e],c2);patch([0 0 1 1-e 0+e 0+e],[0 1 1 1-e 1-e 0+e],c3);plot([0 1 1 0 0],[0 0 1 1 0]);disp('+');
  tansig : neural/Transfer Functions/tansig
  "a{1}" : Outport  InitialOutput=[0;0;0;0;0;0;0;0;0;0]
      mask Display: e = 0.06;c1 = [120 230 180]/255;c2 = ([120 230 180]+0)/(256+128);c3 = ([120 230 180]+128)/(256+128);patch([0 1 1 0],[0 0 1 1],c1);patch([0 1 1 1-e 1-e 0+e],[0 0 1 1-e 0+e 0+e],c2);patch([0 0 1 1-e 0+e 0+e],[0 1 1 1-e 1-e 0+e],c3);plot([0 1 1 0 0],[0 0 1 1 0]);
  wires:
  "p{1}"/1 -> Delays 1/1("p{1}")
  Delays 1/1("pd{1,1}") -> "IW{1,1}"/1("pd{1,1}")
  "IW{1,1}"/1("iz{1,1}") -> netsum/1
  "b{1}"/1 -> netsum/2
  netsum/1 -> tansig/1
  tansig/1 -> "a{1}"/1

== system case2_DCMG_attack_network_detailed_model_R2016/Subsystem3/Feed-Forward Neural Network/Layer 2 ==
  "a{1} " : Inport  PortDimensions=10
      mask Display: e = 0.06;c1 = [120 230 180]/255;c2 = ([120 230 180]+0)/(256+128);c3 = ([120 230 180]+128)/(256+128);patch([0 1 1 0],[0 0 1 1],c1);patch([0 1 1 1-e 1-e 0+e],[0 0 1 1-e 0+e 0+e],c2);patch([0 0 1 1-e 0+e 0+e],[0 1 1 1-e 1-e 0+e],c3);plot([0 1 1 0 0],[0 0 1 1 0]);
  Delays 1 : Subsystem
      mask Display: e = 0.06;c1 = [120 150 230]/255;c2 = ([120 150 230]+0)/383;c3 = ([120 150 230]+128)/383;patch([0 1 1 0],[0 0 1 1],c1);patch([0 1 1 1-e 1-e 0+e],[0 0 1 1-e 0+e 0+e],c2);patch([0 0 1 1-e 0+e 0+e],[0 1 1 1-e 1-e 0+e],c3);plot([0 1 1 0 0],[0 0 1 1 0]);disp('0');
  "LW{2,1}" : Subsystem
      mask Display: e = 0.06;c1 = [120 150 230]/255;c2 = ([120 150 230]+0)/383;c3 = ([120 150 230]+128)/383;patch([0 1 1 0],[0 0 1 1],c1);patch([0 1 1 1-e 1-e 0+e],[0 0 1 1-e 0+e 0+e],c2);patch([0 0 1 1-e 0+e 0+e],[0 1 1 1-e 1-e 0+e],c3);plot([0 1 1 0 0],[0 0 1 1 0]);disp('W');
  "b{2}" : Constant  Value=0.174919756746073906672478415202931500971317291259765625
      mask Display: e = 0.06;c1 = [120 150 230]/255;c2 = ([120 150 230]+0)/383;c3 = ([120 150 230]+128)/383;patch([0 1 1 0],[0 0 1 1],c1);patch([0 1 1 1-e 1-e 0+e],[0 0 1 1-e 0+e 0+e],c2);patch([0 0 1 1-e 0+e 0+e],[0 1 1 1-e 1-e 0+e],c3);plot([0 1 1 0 0],[0 0 1 1 0]);disp('b');
  netsum : Sum  Inputs=2  InputSameDT=on  SaturateOnIntegerOverflow=on  OutDataTypeStr=Inherit: Same as first input
      mask Display: e = 0.06;c1 = [120 150 230]/255;c2 = ([120 150 230]+0)/383;c3 = ([120 150 230]+128)/383;patch([0 1 1 0],[0 0 1 1],c1);patch([0 1 1 1-e 1-e 0+e],[0 0 1 1-e 0+e 0+e],c2);patch([0 0 1 1-e 0+e 0+e],[0 1 1 1-e 1-e 0+e],c3);plot([0 1 1 0 0],[0 0 1 1 0]);disp('+');
  purelin : neural/Transfer Functions/purelin
  "a{2}" : Outport  InitialOutput=0
      mask Display: e = 0.06;c1 = [120 230 180]/255;c2 = ([120 230 180]+0)/(256+128);c3 = ([120 230 180]+128)/(256+128);patch([0 1 1 0],[0 0 1 1],c1);patch([0 1 1 1-e 1-e 0+e],[0 0 1 1-e 0+e 0+e],c2);patch([0 0 1 1-e 0+e 0+e],[0 1 1 1-e 1-e 0+e],c3);plot([0 1 1 0 0],[0 0 1 1 0]);
  wires:
  "a{1} "/1 -> Delays 1/1("p{2}")
  Delays 1/1("pd{2,1}") -> "LW{2,1}"/1("ad{2,1}")
  "LW{2,1}"/1("lz{2,1}") -> netsum/1
  "b{2}"/1 -> netsum/2
  netsum/1 -> purelin/1
  purelin/1 -> "a{2}"/1

== system case2_DCMG_attack_network_detailed_model_R2016/Subsystem3/Feed-Forward Neural Network/Process Input 1 ==
  x : Inport  PortDimensions=8
      mask Display: e = 0.06;c1 = [120 230 180]/255;c2 = ([120 230 180]+0)/(256+128);c3 = ([120 230 180]+128)/(256+128);patch([0 1 1 0],[0 0 1 1],c1);patch([0 1 1 1-e 1-e 0+e],[0 0 1 1-e 0+e 0+e],c2);patch([0 0 1 1-e 0+e 0+e],[0 1 1 1-e 1-e 0+e],c3);plot([0 1 1 0 0],[0 0 1 1 0]);
  mapminmax : neural/Processing Functions/mapminmax  xmin=[0.527531554607323149852504684532;0.527531554607323149852504684532;0.516317459888330221318142321252;0.516317459888330221318142321252;125.052286639662767697700473946;125.052286639662767697700473946;125.098356428801508855030988343;125.098356428801508855030988343]  xmax=[105.803676226220090939023066312;105.803676226220090939023066312;103.503625220714923216291936114;103.503625220714923216291936114;177.862229771129563005160889588;177.862229771129563005160889588;187.062566790448443043715087697;187.062566790448443043715087697]  ymin=-1  ymax=1
  p : Outport  PortDimensions=8
      mask Display: e = 0.06;c1 = [120 230 180]/255;c2 = ([120 230 180]+0)/(256+128);c3 = ([120 230 180]+128)/(256+128);patch([0 1 1 0],[0 0 1 1],c1);patch([0 1 1 1-e 1-e 0+e],[0 0 1 1-e 0+e 0+e],c2);patch([0 0 1 1-e 0+e 0+e],[0 1 1 1-e 1-e 0+e],c3);plot([0 1 1 0 0],[0 0 1 1 0]);
  wires:
  x/1 -> mapminmax/1
  mapminmax/1 -> p/1

== system case2_DCMG_attack_network_detailed_model_R2016/Subsystem3/Feed-Forward Neural Network/Process Output 1 ==
  a : Inport  PortDimensions=1
      mask Display: e = 0.06;c1 = [120 230 180]/255;c2 = ([120 230 180]+0)/(256+128);c3 = ([120 230 180]+128)/(256+128);patch([0 1 1 0],[0 0 1 1],c1);patch([0 1 1 1-e 1-e 0+e],[0 0 1 1-e 0+e 0+e],c2);patch([0 0 1 1-e 0+e 0+e],[0 1 1 1-e 1-e 0+e],c3);plot([0 1 1 0 0],[0 0 1 1 0]);
  mapminmax_reverse : neural/Processing Functions/mapminmax_reverse  xmin=97.057360749590500859085295815  xmax=168.89908936871114519817638211  ymin=-1  ymax=1
  y : Outport  PortDimensions=1
      mask Display: e = 0.06;c1 = [120 230 180]/255;c2 = ([120 230 180]+0)/(256+128);c3 = ([120 230 180]+128)/(256+128);patch([0 1 1 0],[0 0 1 1],c1);patch([0 1 1 1-e 1-e 0+e],[0 0 1 1-e 0+e 0+e],c2);patch([0 0 1 1-e 0+e 0+e],[0 1 1 1-e 1-e 0+e],c3);plot([0 1 1 0 0],[0 0 1 1 0]);
  wires:
  a/1 -> mapminmax_reverse/1
  mapminmax_reverse/1 -> y/1

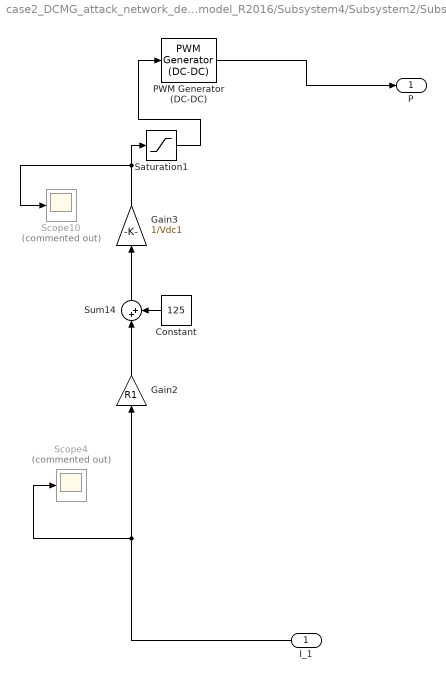
== system case2_DCMG_attack_network_detailed_model_R2016/Subsystem4/Subsystem2/Subsystem ==
  I_1 : Inport
  Constant : Constant  Value=125  SampleTime=Ts
  Gain2 : Gain  Gain=R1
  Gain3 : Gain  Gain=1/Vdc1
  PWM Generator (DC-DC) : powerlib_meascontrol/Pulse & Signal Generators/PWM Generator (DC-DC)  Fsw=5000  Ts=Ts
  Saturation1 : Saturate  UpperLimit=1  LowerLimit=0
  Scope10 : Scope  Commented=on
  Scope4 : Scope  Commented=on
  Sum14 : Sum  Inputs=|++
  P : Outport
  wires:
  I_1/1 -> Scope4/1, Gain2/1
  Sum14/1 -> Gain3/1
  Gain3/1 -> Saturation1/1, Scope10/1
  Constant/1 -> Sum14/2
  Gain2/1 -> Sum14/1
  Saturation1/1 -> PWM Generator (DC-DC)/1
  PWM Generator (DC-DC)/1 -> P/1

== system case2_DCMG_attack_network_detailed_model_R2016/Subsystem4/Subsystem2/Subsystem1 ==
  I_2 : Inport
  Constant1 : Constant  Value=125  SampleTime=Ts
  Gain4 : Gain  Gain=R2
  Gain5 : Gain  Gain=1/Vdc2
  Saturation2 : Saturate  UpperLimit=1  LowerLimit=0
  Sum15 : Sum  Inputs=|++
  Out1 : Outport
  wires:
  Gain4/1 -> Sum15/1
  Constant1/1 -> Sum15/2
  Saturation2/1 -> Out1/1
  Gain5/1 -> Saturation2/1
  Sum15/1 -> Gain5/1
  I_2/1 -> Gain4/1

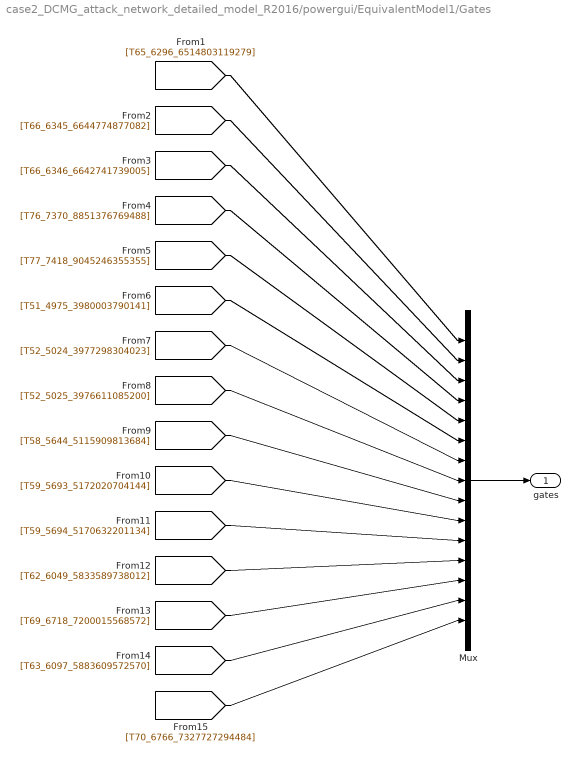
== system case2_DCMG_attack_network_detailed_model_R2016/powergui/EquivalentModel1/Gates ==
  Mux : Mux  Inputs=[1 1 1 1 1 1 1 1 1 1 1 1 1 1 1]
  gates : Outport
  wires:
  Mux/1 -> gates/1
  [T65_6296_6514803119279] -> Mux/1
  [T66_6345_6644774877082] -> Mux/2
  [T66_6346_6642741739005] -> Mux/3
  [T76_7370_8851376769488] -> Mux/4
  [T77_7418_9045246355355] -> Mux/5
  [T51_4975_3980003790141] -> Mux/6
  [T52_5024_3977298304023] -> Mux/7
  [T52_5025_3976611085200] -> Mux/8
  [T58_5644_5115909813684] -> Mux/9
  [T59_5693_5172020704144] -> Mux/10
  [T59_5694_5170632201134] -> Mux/11
  [T62_6049_5833589738012] -> Mux/12
  [T69_6718_7200015568572] -> Mux/13
  [T63_6097_5883609572570] -> Mux/14
  [T70_6766_7327727294484] -> Mux/15

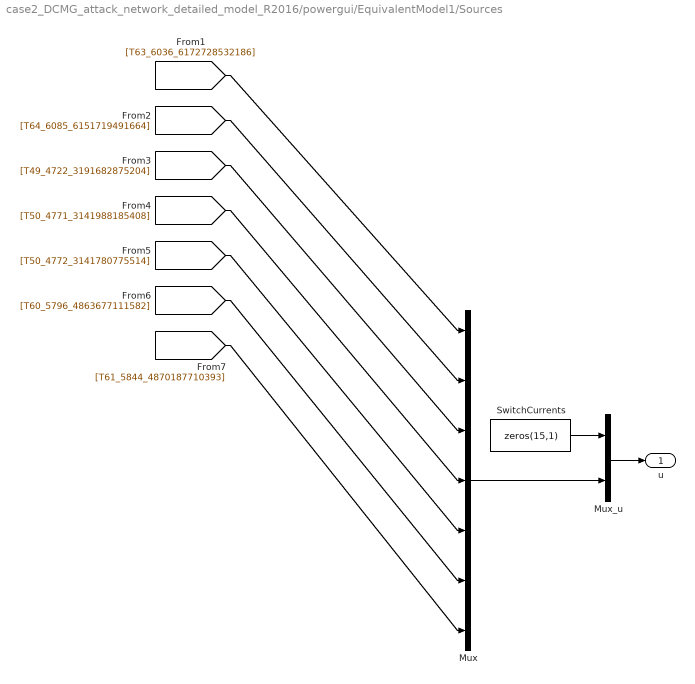
== system case2_DCMG_attack_network_detailed_model_R2016/powergui/EquivalentModel1/Sources ==
  Mux : Mux  Inputs=[1 1 1 1 1 1 1]
  Mux_u : Mux  Inputs=[15 7]
  SwitchCurrents : Constant  Value=zeros(15,1)
  u : Outport
  wires:
  Mux_u/1 -> u/1
  SwitchCurrents/1 -> Mux_u/1
  Mux/1 -> Mux_u/2
  [T63_6036_6172728532186] -> Mux/1
  [T64_6085_6151719491664] -> Mux/2
  [T49_4722_3191682875204] -> Mux/3
  [T50_4771_3141988185408] -> Mux/4
  [T50_4772_3141780775514] -> Mux/5
  [T60_5796_4863677111582] -> Mux/6
  [T61_5844_4870187710393] -> Mux/7

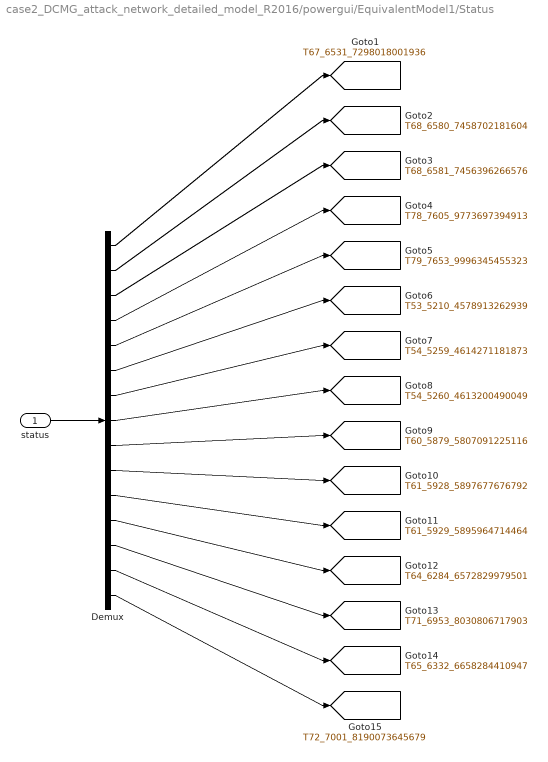
== system case2_DCMG_attack_network_detailed_model_R2016/powergui/EquivalentModel1/Status ==
  status : Inport
  Demux : Demux  Outputs=[1 1 1 1 1 1 1 1 1 1 1 1 1 1 1]
  tag scope: T53_5210_4578913262939=global, T54_5259_4614271181873=global, T54_5260_4613200490049=global, T60_5879_5807091225116=global, T61_5928_5897677676792=global, T61_5929_5895964714464=global, T64_6284_6572829979501=global, T65_6332_6658284410947=global, T67_6531_7298018001936=global, T68_6580_7458702181604=global, T68_6581_7456396266576=global, T71_6953_8030806717903=global, T72_7001_8190073645679=global, T78_7605_9773697394913=global, T79_7653_9996345455323=global
  wires:
  status/1 -> Demux/1
  Demux/1 -> [T67_6531_7298018001936]
  Demux/2 -> [T68_6580_7458702181604]
  Demux/3 -> [T68_6581_7456396266576]
  Demux/4 -> [T78_7605_9773697394913]
  Demux/5 -> [T79_7653_9996345455323]
  Demux/6 -> [T53_5210_4578913262939]
  Demux/7 -> [T54_5259_4614271181873]
  Demux/8 -> [T54_5260_4613200490049]
  Demux/9 -> [T60_5879_5807091225116]
  Demux/10 -> [T61_5928_5897677676792]
  Demux/11 -> [T61_5929_5895964714464]
  Demux/12 -> [T64_6284_6572829979501]
  Demux/13 -> [T71_6953_8030806717903]
  Demux/14 -> [T65_6332_6658284410947]
  Demux/15 -> [T72_7001_8190073645679]

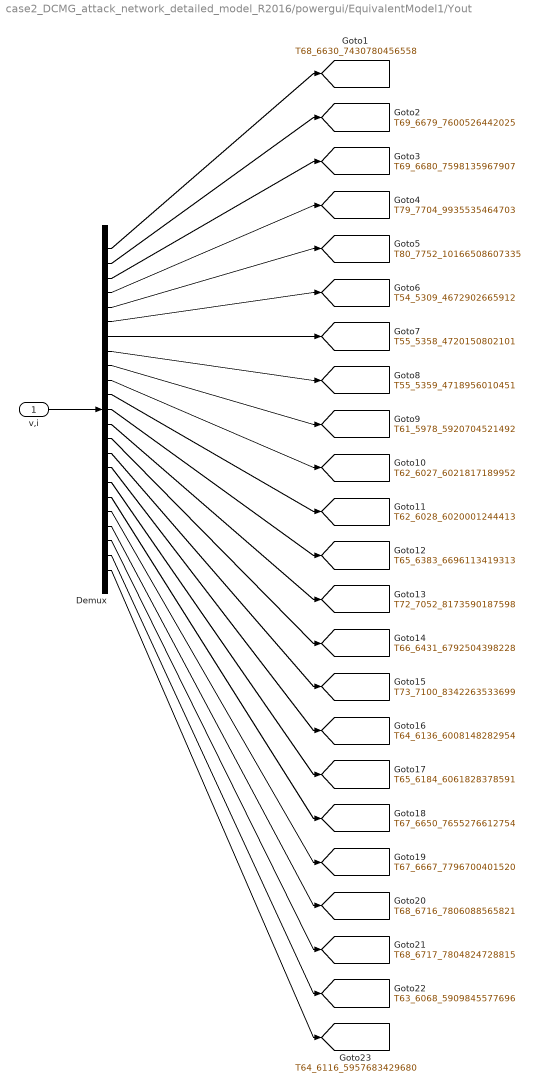
== system case2_DCMG_attack_network_detailed_model_R2016/powergui/EquivalentModel1/Yout ==
  v,i : Inport
  Demux : Demux  Outputs=[1 1 1 1 1 1 1 1 1 1 1 1 1 1 1 1 1 1 1 1 1 1 1]
  tag scope: T54_5309_4672902665912=global, T55_5358_4720150802101=global, T55_5359_4718956010451=global, T61_5978_5920704521492=global, T62_6027_6021817189952=global, T62_6028_6020001244413=global, T63_6068_5909845577696=global, T64_6116_5957683429680=global, T64_6136_6008148282954=global, T65_6184_6061828378591=global, T65_6383_6696113419313=global, T66_6431_6792504398228=global, T67_6650_7655276612754=global, T67_6667_7796700401520=global, T68_6630_7430780456558=global, T68_6716_7806088565821=global, T68_6717_7804824728815=global, T69_6679_7600526442025=global, T69_6680_7598135967907=global, T72_7052_8173590187598=global, T73_7100_8342263533699=global, T79_7704_9935535464703=global, T80_7752_10166508607335=global
  wires:
  v,i/1 -> Demux/1
  Demux/1 -> [T68_6630_7430780456558]
  Demux/2 -> [T69_6679_7600526442025]
  Demux/3 -> [T69_6680_7598135967907]
  Demux/4 -> [T79_7704_9935535464703]
  Demux/5 -> [T80_7752_10166508607335]
  Demux/6 -> [T54_5309_4672902665912]
  Demux/7 -> [T55_5358_4720150802101]
  Demux/8 -> [T55_5359_4718956010451]
  Demux/9 -> [T61_5978_5920704521492]
  Demux/10 -> [T62_6027_6021817189952]
  Demux/11 -> [T62_6028_6020001244413]
  Demux/12 -> [T65_6383_6696113419313]
  Demux/13 -> [T72_7052_8173590187598]
  Demux/14 -> [T66_6431_6792504398228]
  Demux/15 -> [T73_7100_8342263533699]
  Demux/16 -> [T64_6136_6008148282954]
  Demux/17 -> [T65_6184_6061828378591]
  Demux/18 -> [T67_6650_7655276612754]
  Demux/19 -> [T67_6667_7796700401520]
  Demux/20 -> [T68_6716_7806088565821]
  Demux/21 -> [T68_6717_7804824728815]
  Demux/22 -> [T63_6068_5909845577696]
  Demux/23 -> [T64_6116_5957683429680]

== system case2_DCMG_attack_network_detailed_model_R2016/Subsystem3/Feed-Forward Neural Network/Layer 1/Delays 1 ==
  "p{1}" : Inport  PortDimensions=8
      mask Display: e = 0.06;c1 = [120 230 180]/255;c2 = ([120 230 180]+0)/(256+128);c3 = ([120 230 180]+128)/(256+128);patch([0 1 1 0],[0 0 1 1],c1);patch([0 1 1 1-e 1-e 0+e],[0 0 1 1-e 0+e 0+e],c2);patch([0 0 1 1-e 0+e 0+e],[0 1 1 1-e 1-e 0+e],c3);plot([0 1 1 0 0],[0 0 1 1 0]);
  mux : Mux  Inputs=1
      mask Display: e = 0.06;c1 = [120 150 230]/255;c2 = ([120 150 230]+0)/383;c3 = ([120 150 230]+128)/383;patch([0 1 1 0],[0 0 1 1],c1);patch([0 1 1 1-e 1-e 0+e],[0 0 1 1-e 0+e 0+e],c2);patch([0 0 1 1-e 0+e 0+e],[0 1 1 1-e 1-e 0+e],c3);plot([0 1 1 0 0],[0 0 1 1 0]);disp('Mux')
  "pd{1,1}" : Outport
      mask Display: e = 0.06;c1 = [120 230 180]/255;c2 = ([120 230 180]+0)/(256+128);c3 = ([120 230 180]+128)/(256+128);patch([0 1 1 0],[0 0 1 1],c1);patch([0 1 1 1-e 1-e 0+e],[0 0 1 1-e 0+e 0+e],c2);patch([0 0 1 1-e 0+e 0+e],[0 1 1 1-e 1-e 0+e],c3);plot([0 1 1 0 0],[0 0 1 1 0]);
  wires:
  "p{1}"/1 -> mux/1
  mux/1 -> "pd{1,1}"/1
